simulink model "MotionControl"  (R2020a)
settings: Solver=VariableStepAuto  StartTime=0.0  StopTime=10.0  RelTol=1e-3
settings Model: DataDictionary=RobotDD.sldd  Creator=Sony  LastModifiedBy=Sony

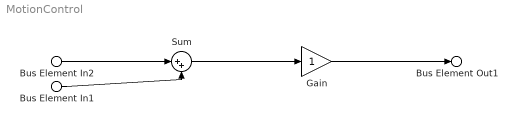
== system MotionControl ==
  Bus Element In2 : Inport  PortName=Sensors Data
  Bus Element In1 : Inport  Port=2  PortName=Target Position
  Gain : Gain
  Sum : Sum  Inputs=|++
  Bus Element Out1 : Outport  PortName=Command
  wires:
  Bus Element In2/1 -> Sum/1
  Bus Element In1/1 -> Sum/2
  Sum/1 -> Gain/1
  Gain/1 -> Bus Element Out1/1
